simulink model "Universal_Convert_2"  (R2025a)
settings: Solver=VariableStepAuto  StartTime=0.0  StopTime=10.0  RelTol=1e-3
settings Model: LastModifiedBy=Johan

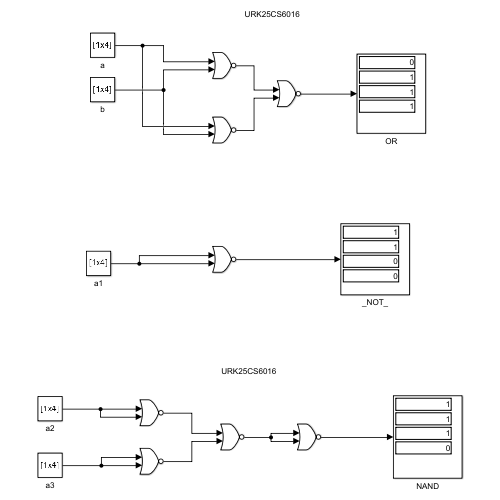
[thumbnail: Simulink's stored preview of the top-level diagram]
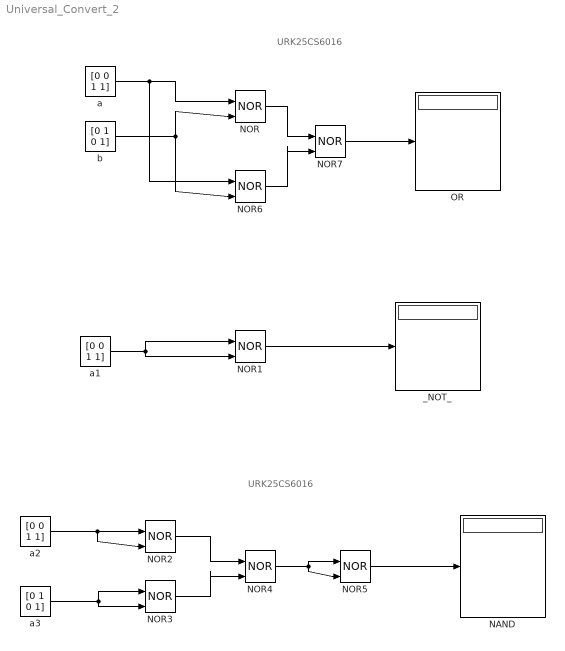
== system Universal_Convert_2 ==
  note: URK25CS6016
  note: URK25CS6016
  NAND : Display
  NOR{,1..7} (8 alike) : Logic  Operator=NOR  IconShape=distinctive  AllPortsSameDT=off  OutDataTypeStr=boolean
  OR : Display
  _NOT_ : Display
  a : Constant  Value=[0 0 1 1]
  a1 : Constant  Value=[0 0 1 1]
  a2 : Constant  Value=[0 0 1 1]
  a3 : Constant  Value=[0 1 0 1]
  b : Constant  Value=[0 1 0 1]
  wires:
  NOR1/1 -> _NOT_/1
  a1/1 -> NOR1/1, NOR1/2
  a2/1 -> NOR2/2, NOR2/1
  a3/1 -> NOR3/1, NOR3/2
  NOR2/1 -> NOR4/1
  NOR3/1 -> NOR4/2
  NOR4/1 -> NOR5/2, NOR5/1
  NOR5/1 -> NAND/1
  NOR/1 -> NOR7/1
  NOR6/1 -> NOR7/2
  NOR7/1 -> OR/1
  a/1 -> NOR6/1, NOR/1
  b/1 -> NOR6/2, NOR/2
